simulink model "Sensores_piero"  (R2022b)
settings: Solver=VariableStepAuto  StartTime=0.0  StopTime=10.0  RelTol=1e-3
libraries: arduinolib x2
settings Model: Creator=marqu  LastModifiedBy=marqu

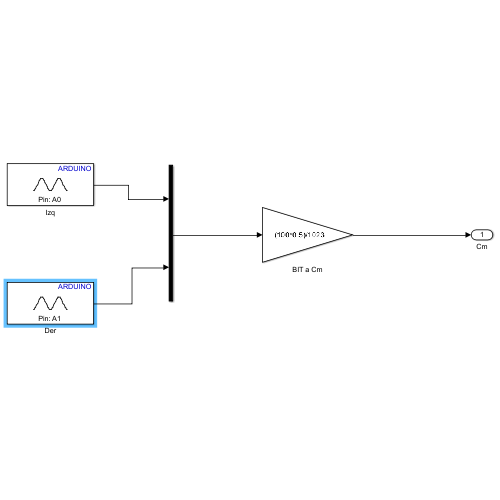
[thumbnail: Simulink's stored preview of the top-level diagram]
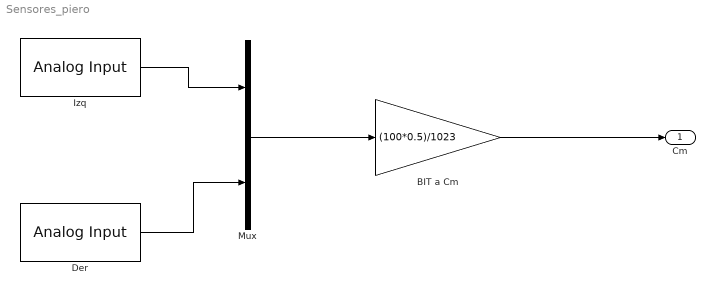
== system Sensores_piero ==
  BIT a Cm : Gain  Gain=(100*0.5)/1023
  Der : arduinolib/Analog Input  pinNumber=1  ReadResultsOnly=off  ConversionTriggerSource=Software  ExternalTriggerType=uint32( 0 )  OutputDataType=uint16  EnableConversionCompleteNotify=off  EnableOuputStatus=off  SampleTime=-1  blockPlatform=arduino
  Izq : arduinolib/Analog Input  pinNumber=0  ReadResultsOnly=off  ConversionTriggerSource=Software  ExternalTriggerType=uint32( 0 )  OutputDataType=uint16  EnableConversionCompleteNotify=off  EnableOuputStatus=off  SampleTime=-1  blockPlatform=arduino
  Mux : Mux  Inputs=2
  Cm : Outport
  wires:
  Izq/1 -> Mux/1
  Der/1 -> Mux/2
  Mux/1 -> BIT a Cm/1
  BIT a Cm/1 -> Cm/1
